simulink library "Navigation_KF_Lib"  (R2016a)
settings: Solver=ode45  StartTime=0.0  StopTime=10.0  RelTol=1e-3
undefined symbols (not defined in the file or in its folder): Accel_Calib_Gain, Accel_Calib_Offset, Mag_Calib_Gain_Vector, Mag_Calib_Offset_Vector
libraries: simulink x5, vrlib x4, aerolibtransform2 x2, aerolibutil x1
(part 1 of 2)
settings Model: Creator=darenlee  LastModifiedBy=sannem
settings DataIOCC: LimitDataPoints=on  SaveFormat=Array
settings DebuggingCC: SolverPrmCheckMsg=warning
settings HardwareCC: ProdBitPerPointer=32  ProdLargestAtomicFloat=None  ProdIntDivRoundTo=Undefined  ProdEndianess=Unspecified  ProdWordSize=32  ProdHWDeviceType=32-bit Generic
settings ModelReferenceCC: PropagateSignalLabelsOutOfModel=off
settings ConfigComp: CovModelRefEnable=Off  CovSFcnEnable=off

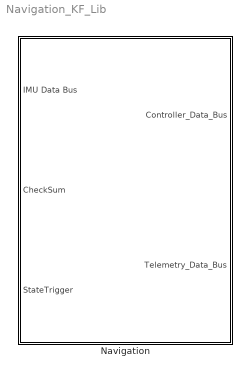
== system Navigation_KF_Lib ==
  Navigation : Subsystem
      mask DialogControl DescTextVar Prompt: Kalman Filter Navigation Implementation

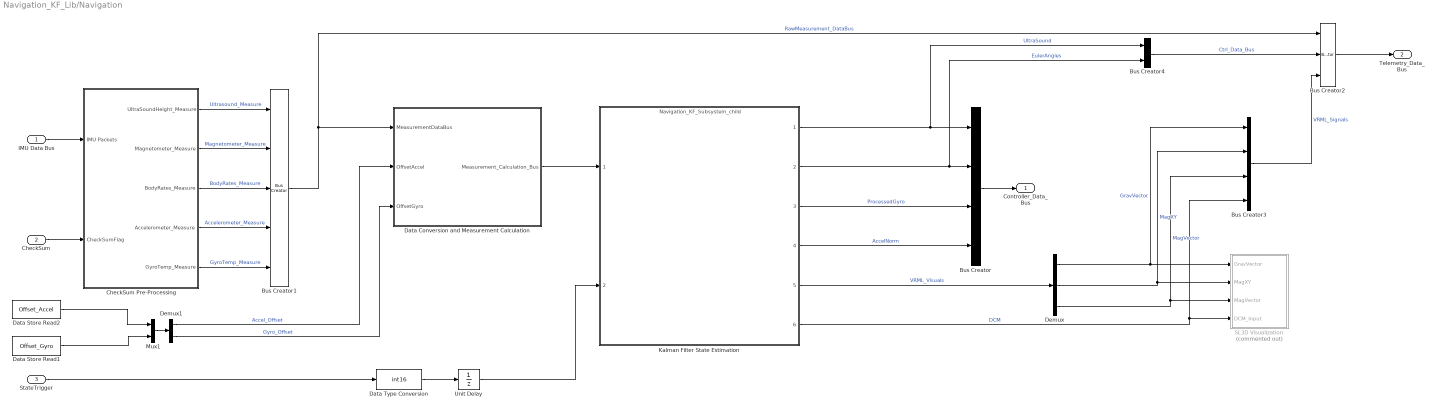
== system Navigation_KF_Lib/Navigation ==
  IMU Data Bus : Inport  OutDataTypeStr=Bus: IMU_Packets
  CheckSum : Inport  Port=2
  StateTrigger : Inport  Port=3  OutDataTypeStr=Enum: Drone_StateModeType
  Bus Creator : BusCreator  Inputs=4
  Bus Creator1 : BusCreator  Inputs=5
  Bus Creator2 : BusCreator  Inputs=3
  Bus Creator3 : BusCreator  Inputs=4
  Bus Creator4 : BusCreator  Inputs=2
  CheckSum Pre-Processing : Subsystem  TreatAsAtomicUnit=on
      settings: RTWSystemCode=Inline
  Data Conversion and Measurement Calculation : Subsystem
  Data Store Read1 : DataStoreRead  DataStoreName=Offset_Gyro
  Data Store Read2 : DataStoreRead  DataStoreName=Offset_Accel
  Data Type Conversion : DataTypeConversion  OutDataTypeStr=int16
  Demux : Demux  Outputs=[3 3 3]
  Demux1 : Demux  Outputs=[2 3]
  Kalman Filter State Estimation : ModelReference  ModelNameDialog=Navigation_KF_Subsystem_child.slx  SimulationMode=Normal  ModelReferenceVersion=1.56
  Mux1 : Mux  Inputs=2
  SL3D Visualization : Subsystem  Commented=on
  Unit Delay : UnitDelay  SampleTime=-1
  Controller_Data_Bus : Outport
  Telemetry_Data_Bus : Outport  Port=2
  wires:
  Bus Creator4/1 -> Bus Creator2/2  "Ctrl_Data_Bus"
  Demux/2 -> SL3D Visualization/2(MagXY), Bus Creator3/2  "MagXY"
  Bus Creator3/1 -> Bus Creator2/3  "VRML_Signals"
  Bus Creator2/1 -> Telemetry_Data_Bus/1
  Data Store Read1/1 -> Mux1/2
  Data Store Read2/1 -> Mux1/1
  Kalman Filter State Estimation/5 -> Demux/1  "VRML_Visuals"
  Kalman Filter State Estimation/2 -> Bus Creator/2, Bus Creator4/2  "EulerAngles"
  Bus Creator/1 -> Controller_Data_Bus/1
  Demux/3 -> SL3D Visualization/3(MagVector), Bus Creator3/3  "MagVector"
  Demux/1 -> SL3D Visualization/1(GravVector), Bus Creator3/1  "GravVector"
  Kalman Filter State Estimation/1 -> Bus Creator/1, Bus Creator4/1  "UltraSound"
  Kalman Filter State Estimation/6 -> SL3D Visualization/4(DCM_Input), Bus Creator3/4  "DCM"
  Data Type Conversion/1 -> Unit Delay/1
  Unit Delay/1 -> Kalman Filter State Estimation/2
  IMU Data Bus/1 -> CheckSum Pre-Processing/1(IMU Packets)
  CheckSum/1 -> CheckSum Pre-Processing/2(CheckSumFlag)
  CheckSum Pre-Processing/1(UltraSoundHeight_Measure) -> Bus Creator1/1  "Ultrasound_Measure"
  CheckSum Pre-Processing/2(Magnetometer_Measure) -> Bus Creator1/2  "Magnetometer_Measure"
  CheckSum Pre-Processing/3(BodyRates_Measure) -> Bus Creator1/3  "BodyRates_Measure"
  CheckSum Pre-Processing/4(Accelerometer_Measure) -> Bus Creator1/4  "Accelerometer_Measure"
  CheckSum Pre-Processing/5(GyroTemp_Measure) -> Bus Creator1/5  "GyroTemp_Measure"
  Bus Creator1/1 -> Data Conversion and Measurement Calculation/1(MeasurementDataBus), Bus Creator2/1  "RawMeasurement_DataBus"
  Mux1/1 -> Demux1/1
  Demux1/1 -> Data Conversion and Measurement Calculation/2(OffsetAccel)  "Accel_Offset"
  Demux1/2 -> Data Conversion and Measurement Calculation/3(OffsetGyro)  "Gyro_Offset"
  StateTrigger/1 -> Data Type Conversion/1
  Data Conversion and Measurement Calculation/1(Measurement_Calculation_Bus) -> Kalman Filter State Estimation/1
  Kalman Filter State Estimation/3 -> Bus Creator/3  "ProcessedGyro"
  Kalman Filter State Estimation/4 -> Bus Creator/4  "AccelNorm"

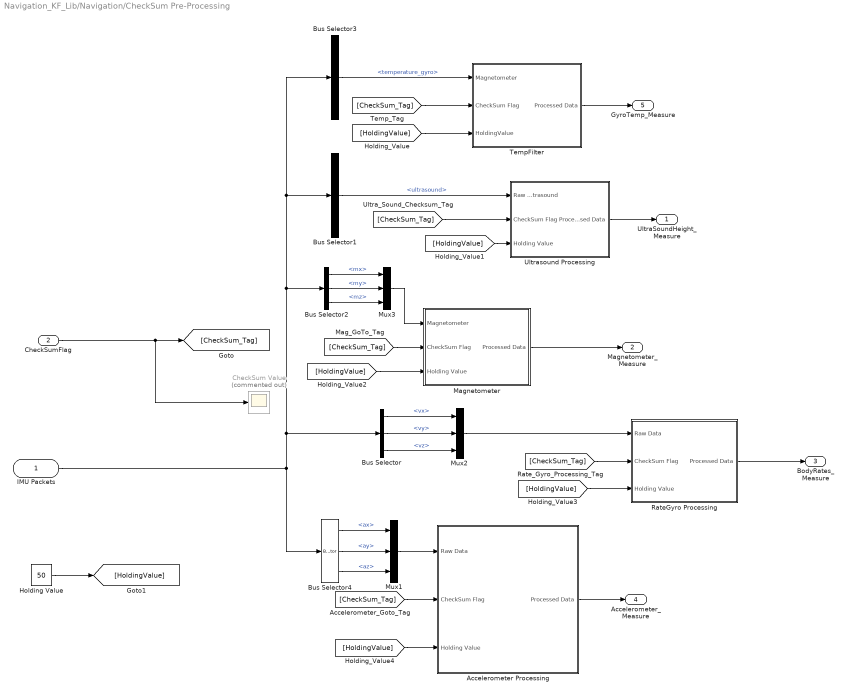
== system Navigation_KF_Lib/Navigation/CheckSum Pre-Processing ==
  IMU Packets : Inport
  CheckSumFlag : Inport  Port=2
  Accelerometer Processing : Subsystem
  Bus Selector : BusSelector  OutputSignals=vx,vy,vz
  Bus Selector1 : BusSelector  OutputSignals=ultrasound
  Bus Selector2 : BusSelector  OutputSignals=mx,my,mz
  Bus Selector3 : BusSelector  OutputSignals=temperature_gyro
  Bus Selector4 : BusSelector  OutputSignals=ax,ay,az
  CheckSum Value : Scope  Commented=on
  Holding Value : Constant  Value=50
  Magnetometer : Subsystem
  Mux1 : Mux  Inputs=3
  Mux2 : Mux  Inputs=3
  Mux3 : Mux  Inputs=3
  RateGyro Processing : Subsystem
  TempFilter : Subsystem
  Ultrasound Processing : Subsystem
  UltraSoundHeight_Measure : Outport
  Magnetometer_Measure : Outport  Port=2
  BodyRates_Measure : Outport  Port=3
  Accelerometer_Measure : Outport  Port=4
  GyroTemp_Measure : Outport  Port=5
  wires:
  Bus Selector1/1 -> Ultrasound Processing/1(Raw Ultrasound)  "<ultrasound>"
  CheckSumFlag/1 -> [CheckSum_Tag], CheckSum Value/1
  IMU Packets/1 -> Bus Selector/1, Bus Selector3/1, Bus Selector1/1, Bus Selector2/1, Bus Selector4/1
  Bus Selector4/1 -> Mux1/1  "<ax>"
  Bus Selector4/2 -> Mux1/2  "<ay>"
  Bus Selector4/3 -> Mux1/3  "<az>"
  Mux1/1 -> Accelerometer Processing/1(Raw Data)
  [CheckSum_Tag] -> Ultrasound Processing/2(CheckSum Flag)
  Accelerometer Processing/1(Processed Data) -> Accelerometer_Measure/1
  Mux2/1 -> RateGyro Processing/1(Raw Data)
  [CheckSum_Tag] -> RateGyro Processing/2(CheckSum Flag)
  RateGyro Processing/1(Processed Data) -> BodyRates_Measure/1
  Bus Selector2/1 -> Mux3/1  "<mx>"
  Bus Selector2/2 -> Mux3/2  "<my>"
  Bus Selector2/3 -> Mux3/3  "<mz>"
  [CheckSum_Tag] -> Magnetometer/2(CheckSum Flag)
  Magnetometer/1(Processed Data) -> Magnetometer_Measure/1
  [CheckSum_Tag] -> Accelerometer Processing/2(CheckSum Flag)
  Ultrasound Processing/1(Processed Data) -> UltraSoundHeight_Measure/1
  Bus Selector/1 -> Mux2/1  "<vx>"
  Bus Selector/2 -> Mux2/2  "<vy>"
  Bus Selector/3 -> Mux2/3  "<vz>"
  Bus Selector3/1 -> TempFilter/1(Magnetometer)  "<temperature_gyro>"
  TempFilter/1(Processed Data) -> GyroTemp_Measure/1
  [CheckSum_Tag] -> TempFilter/2(CheckSum Flag)
  [HoldingValue] -> TempFilter/3(HoldingValue)
  [HoldingValue] -> Ultrasound Processing/3(Holding Value)
  [HoldingValue] -> Magnetometer/3(Holding Value)
  [HoldingValue] -> RateGyro Processing/3(Holding Value)
  [HoldingValue] -> Accelerometer Processing/3(Holding Value)
  Holding Value/1 -> [HoldingValue]
  Mux3/1 -> Magnetometer/1(Magnetometer)

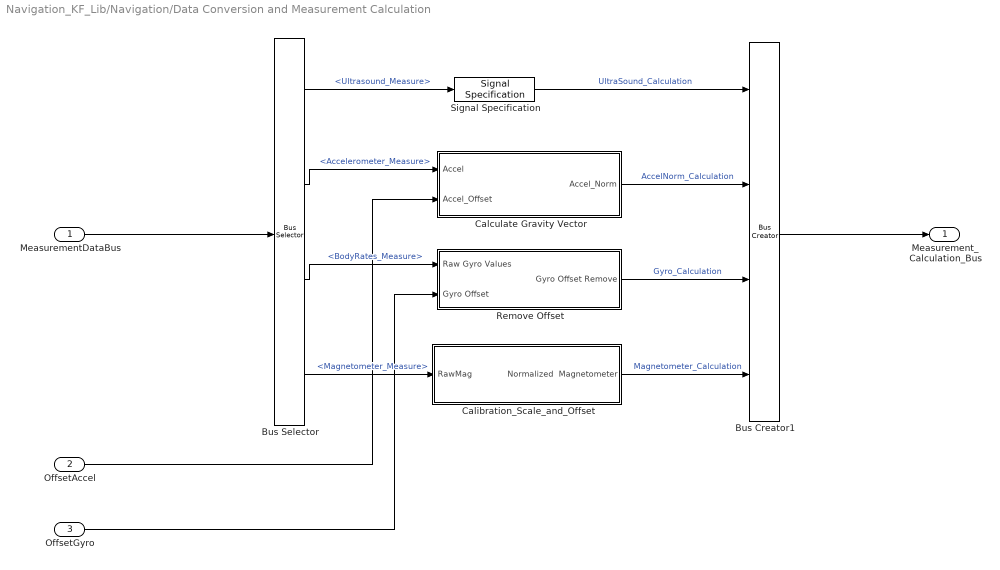
== system Navigation_KF_Lib/Navigation/Data Conversion and Measurement Calculation ==
  MeasurementDataBus : Inport
  OffsetAccel : Inport  Port=2
  OffsetGyro : Inport  Port=3
  Bus Creator1 : BusCreator  Inputs=4
  Bus Selector : BusSelector  OutputSignals=Ultrasound_Measure,Accelerometer_Measure,BodyRates_Measure,Magnetometer_Measure
  Calculate Gravity Vector : Subsystem
  Calibration_Scale_and_Offset : Subsystem
  Remove Offset : Subsystem
  Signal Specification : SignalSpecification
  Measurement_Calculation_Bus : Outport
  wires:
  Bus Selector/2 -> Calculate Gravity Vector/1(Accel)  "<Accelerometer_Measure>"
  Bus Creator1/1 -> Measurement_Calculation_Bus/1
  Calculate Gravity Vector/1(Accel_Norm) -> Bus Creator1/2  "AccelNorm_Calculation"
  Signal Specification/1 -> Bus Creator1/1  "UltraSound_Calculation"
  Remove Offset/1(Gyro Offset Remove) -> Bus Creator1/3  "Gyro_Calculation"
  Calibration_Scale_and_Offset/1(Normalized  Magnetometer) -> Bus Creator1/4  "Magnetometer_Calculation"
  Bus Selector/1 -> Signal Specification/1  "<Ultrasound_Measure>"
  Bus Selector/3 -> Remove Offset/1(Raw Gyro Values)  "<BodyRates_Measure>"
  OffsetGyro/1 -> Remove Offset/2(Gyro Offset)
  OffsetAccel/1 -> Calculate Gravity Vector/2(Accel_Offset)
  Bus Selector/4 -> Calibration_Scale_and_Offset/1(RawMag)  "<Magnetometer_Measure>"
  MeasurementDataBus/1 -> Bus Selector/1

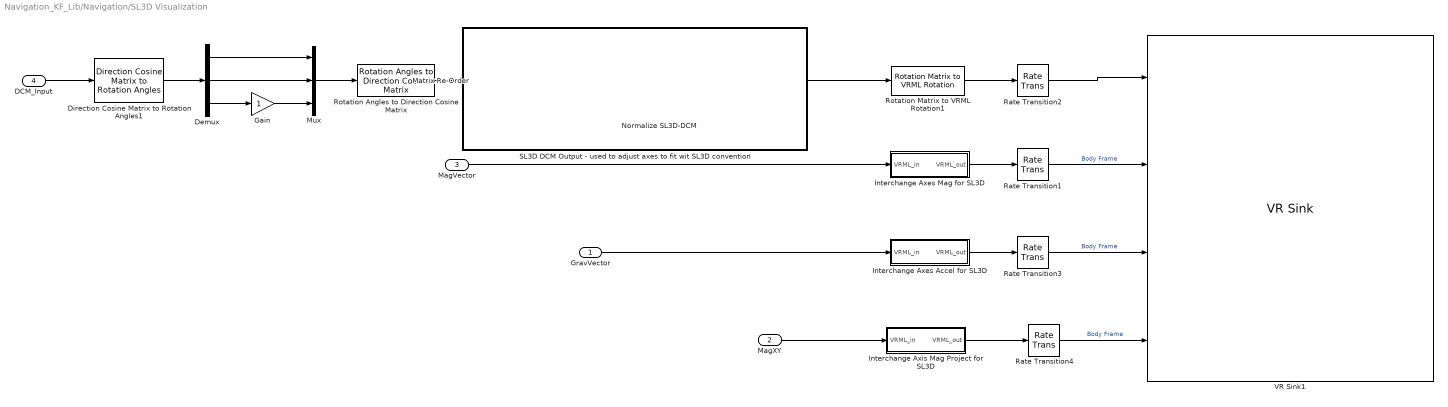
== system Navigation_KF_Lib/Navigation/SL3D Visualization ==
  GravVector : Inport
  MagXY : Inport  Port=2
  MagVector : Inport  Port=3
  DCM_Input : Inport  Port=4
  Demux : Demux  Outputs=3
  Direction Cosine Matrix to Rotation Angles1 : aerolibtransform2/Direction Cosine Matrix to Rotation Angles  rotationOrder=XYZ  lim=ZeroR3
      settings: AttributesFormatString=Rotation Order: %<rotationOrder>
  Gain : Gain  OutDataTypeStr=Inherit: Same as input
  "Interchange Axes Accel for SL3D " : Subsystem
  "Interchange Axes Mag for SL3D " : Subsystem
  Interchange Axis Mag Project for SL3D : Subsystem
  Matrix Re-Order : MATLAB Function  TreatAsAtomicUnit=on
  Mux : Mux  Inputs=3
  Normalize SL3D-DCM : Subsystem  TreatAsAtomicUnit=on
  Rate Transition{1..4} (4 alike) : RateTransition
  Rotation Angles to Direction Cosine Matrix : aerolibtransform2/Rotation Angles to Direction Cosine Matrix  rotationOrder=XYZ
  Rotation Matrix to VRML Rotation1 : vrlib/Utilities/Rotation Matrix to VRML Rotation  maxzero=1e-12
  SL3D DCM Output - used to adjust axes to fit wit SL3D convention : Subsystem
  VR Sink1 : vrlib/VR Sink  InstantiateOnLoad=on  SampleTime=0.02  ViewEnable=on  RemoteChange=off  RemoteView=off  FieldsWritten=Plane.rotation.4.1.1.double#mag_point.translation.3.1.1.double#grav_point.translation.3.1.1.double#mag_projection_point.translation.3.1.1.double  WorldFileName=vrml8_grav_2.WRL  AutoView=off  VideoDimensions=[]  AllowVariableSize=off
  wires:
  Rotation Matrix to VRML Rotation1/1 -> Rate Transition2/1
  "Interchange Axes Accel for SL3D "/1(VRML_out) -> Rate Transition3/1
  DCM_Input/1 -> Direction Cosine Matrix to Rotation Angles1/1
  GravVector/1 -> "Interchange Axes Accel for SL3D "/1(VRML_in)
  Matrix Re-Order/1(M_out) -> Normalize SL3D-DCM/1(DCM)
  Normalize SL3D-DCM/1(DCM_normalized) -> Rotation Matrix to VRML Rotation1/1
  Direction Cosine Matrix to Rotation Angles1/1 -> Demux/1
  Demux/1 -> Mux/1
  Demux/2 -> Mux/2
  Demux/3 -> Gain/1
  Gain/1 -> Mux/3
  Mux/1 -> Rotation Angles to Direction Cosine Matrix/1
  "Interchange Axes Mag for SL3D "/1(VRML_out) -> Rate Transition1/1
  MagVector/1 -> "Interchange Axes Mag for SL3D "/1(VRML_in)
  Rotation Angles to Direction Cosine Matrix/1 -> Matrix Re-Order/1(M_in)
  Interchange Axis Mag Project for SL3D/1(VRML_out) -> Rate Transition4/1
  Rate Transition4/1 -> VR Sink1/4  "Body Frame"
  Rate Transition3/1 -> VR Sink1/3  "Body Frame"
  Rate Transition1/1 -> VR Sink1/2  "Body Frame"
  Rate Transition2/1 -> VR Sink1/1
  MagXY/1 -> Interchange Axis Mag Project for SL3D/1(VRML_in)

== system Navigation_KF_Lib/Navigation/CheckSum Pre-Processing/Accelerometer Processing ==
  Raw Data : Inport
  CheckSum Flag : Inport  Port=2
  Holding Value : Inport  Port=3
  Calculate Accel Data : Subsystem  Commented=through
  CheckSum Correction : Subsystem
  Processed Data : Outport
  wires:
  CheckSum Flag/1 -> CheckSum Correction/2(CheckSumFlag)
  Raw Data/1 -> Calculate Accel Data/1(Raw Accel Data)
  CheckSum Correction/1(Pre-Processed Height) -> Processed Data/1
  Calculate Accel Data/1(Processed Accel Data) -> CheckSum Correction/1(CalculatedData)
  Holding Value/1 -> CheckSum Correction/3(Holding Value)

== system Navigation_KF_Lib/Navigation/CheckSum Pre-Processing/Magnetometer ==
  Magnetometer : Inport
  CheckSum Flag : Inport  Port=2
  Holding Value : Inport  Port=3
  CheckSum Correction : Subsystem
  Process Raw Mag Data : Subsystem  Commented=through
  Processed Data : Outport
  wires:
  CheckSum Flag/1 -> CheckSum Correction/2(CheckSumFlag)
  CheckSum Correction/1(Pre-Processed Data) -> Processed Data/1
  Magnetometer/1 -> Process Raw Mag Data/1(Magnetometer)
  Process Raw Mag Data/1(ProcessedData) -> CheckSum Correction/1(CalculatedData)
  Holding Value/1 -> CheckSum Correction/3(Holding Value)

== system Navigation_KF_Lib/Navigation/CheckSum Pre-Processing/RateGyro Processing ==
  Raw Data : Inport
  CheckSum Flag : Inport  Port=2
  Holding Value : Inport  Port=3
  CheckSum Correction : Subsystem
  Process Data : Subsystem  Commented=through
  Processed Data : Outport
  wires:
  CheckSum Flag/1 -> CheckSum Correction/2(CheckSumFlag)
  CheckSum Correction/1(Pre-Processed Height) -> Processed Data/1
  Raw Data/1 -> Process Data/1(Raw Data)
  Process Data/1(Processed Data) -> CheckSum Correction/1(CalculatedData)
  Holding Value/1 -> CheckSum Correction/3(Holding Value)

== system Navigation_KF_Lib/Navigation/CheckSum Pre-Processing/TempFilter ==
  Magnetometer : Inport
  CheckSum Flag : Inport  Port=2
  HoldingValue : Inport  Port=3
  CheckSum Correction : Subsystem
  Process Raw Mag Data : Subsystem  Commented=through
  Processed Data : Outport
  wires:
  CheckSum Flag/1 -> CheckSum Correction/2(CheckSumFlag)
  CheckSum Correction/1(Pre-Processed Data) -> Processed Data/1
  Magnetometer/1 -> Process Raw Mag Data/1(Magnetometer)
  Process Raw Mag Data/1(ProcessedData) -> CheckSum Correction/1(CalculatedData)
  HoldingValue/1 -> CheckSum Correction/3(Holding Value)

== system Navigation_KF_Lib/Navigation/CheckSum Pre-Processing/Ultrasound Processing ==
  note: '192.168.1.1' 1 17725
  Raw Ultrasound : Inport
  CheckSum Flag : Inport  Port=2
  Holding Value : Inport  Port=3
  CheckSum Correction : Subsystem
  Data Type Conversion1 : DataTypeConversion
  Delay1 : Delay  DelayLength=1  InitialCondition=0
  Height Calculation : MATLAB Function  TreatAsAtomicUnit=on
  Saturation1 : Saturate  UpperLimit=100e3  LowerLimit=0
  Processed Data : Outport
  wires:
  Delay1/1 -> Height Calculation/2(z_1)
  Data Type Conversion1/1 -> Height Calculation/1(u)
  Height Calculation/2(prev_good_height) -> Delay1/1
  Raw Ultrasound/1 -> Data Type Conversion1/1
  Height Calculation/1(y) -> CheckSum Correction/1(CalculatedData)
  CheckSum Flag/1 -> CheckSum Correction/2(CheckSumFlag)
  CheckSum Correction/1(Pre-Processed Height) -> Saturation1/1
  Saturation1/1 -> Processed Data/1
  Holding Value/1 -> CheckSum Correction/3(Holding Value)

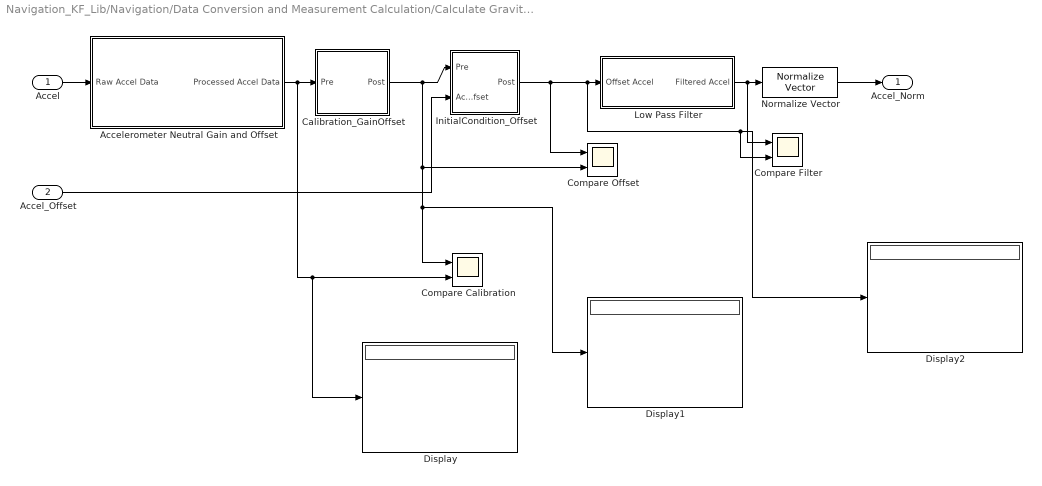
== system Navigation_KF_Lib/Navigation/Data Conversion and Measurement Calculation/Calculate Gravity Vector ==
  Accel : Inport
  Accel_Offset : Inport  Port=2
  Accelerometer Neutral Gain and Offset : Subsystem
  Calibration_GainOffset : Subsystem
  Compare Calibration : Scope  NumInputPorts=2
  Compare Filter : Scope  NumInputPorts=2
  Compare Offset : Scope  NumInputPorts=2
  Display : Display
  Display1 : Display
  Display2 : Display
  InitialCondition_Offset : Subsystem
  Low Pass Filter : Subsystem
  Normalize Vector : vrlib/Utilities/Normalize Vector  maxzero=0
  Accel_Norm : Outport
  wires:
  Normalize Vector/1 -> Accel_Norm/1
  Accel/1 -> Accelerometer Neutral Gain and Offset/1(Raw Accel Data)
  InitialCondition_Offset/1(Post) -> Compare Offset/1, Compare Filter/2, Display2/1, Low Pass Filter/1(Offset Accel)
  Low Pass Filter/1(Filtered Accel) -> Compare Filter/1, Normalize Vector/1
  Calibration_GainOffset/1(Post) -> InitialCondition_Offset/1(Pre), Compare Calibration/1, Display1/1, Compare Offset/2
  Accelerometer Neutral Gain and Offset/1(Processed Accel Data) -> Calibration_GainOffset/1(Pre), Compare Calibration/2, Display/1
  Accel_Offset/1 -> InitialCondition_Offset/2(Accel_Offset)

== system Navigation_KF_Lib/Navigation/Data Conversion and Measurement Calculation/Calibration_Scale_and_Offset ==
  RawMag : Inport
  Normalize Vector : vrlib/Utilities/Normalize Vector  maxzero=0
  Process Raw Mag Data : Subsystem  Variant=on  OverrideUsingVariant=TempVariantA
  Normalized  Magnetometer : Outport
  wires:
  Normalize Vector/1 -> Normalized  Magnetometer/1
  RawMag/1 -> Process Raw Mag Data/1(Magnetometer)
  Process Raw Mag Data/1(MagVector) -> Normalize Vector/1

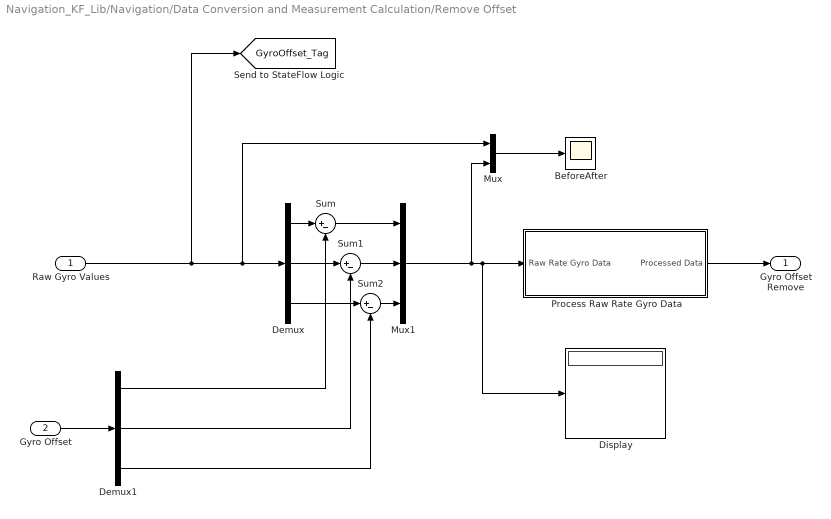
== system Navigation_KF_Lib/Navigation/Data Conversion and Measurement Calculation/Remove Offset ==
  Raw Gyro Values : Inport
  Gyro Offset : Inport  Port=2
  BeforeAfter : Scope
  Demux : Demux  Outputs=3
  Demux1 : Demux  Outputs=3
  Display : Display
  Mux : Mux  Inputs=2
  Mux1 : Mux  Inputs=3
  Process Raw Rate Gyro Data : Subsystem
  Sum : Sum  Inputs=|+-
  Sum1 : Sum  Inputs=|+-
  Sum2 : Sum  Inputs=|+-
  Gyro Offset Remove : Outport
  tag scope: GyroOffset_Tag=global
  wires:
  Sum/1 -> Mux1/1
  Sum2/1 -> Mux1/3
  Demux/3 -> Sum2/1
  Sum1/1 -> Mux1/2
  Demux/1 -> Sum/1
  Demux/2 -> Sum1/1
  Demux1/1 -> Sum/2
  Demux1/2 -> Sum1/2
  Demux1/3 -> Sum2/2
  Mux1/1 -> Mux/2, Display/1, Process Raw Rate Gyro Data/1(Raw Rate Gyro Data)
  Gyro Offset/1 -> Demux1/1
  Raw Gyro Values/1 -> [GyroOffset_Tag], Mux/1, Demux/1
  Mux/1 -> BeforeAfter/1
  Process Raw Rate Gyro Data/1(Processed Data) -> Gyro Offset Remove/1

== system Navigation_KF_Lib/Navigation/SL3D Visualization/Interchange Axes Accel for SL3D  ==
  VRML_in : Inport
  Demux1 : Demux  Outputs=3
  Gain1 : Gain  Gain=3
  Gain2 : Gain
  Gain3 : Gain
  Mux2 : Mux  Inputs=3
  VRML_out : Outport
  wires:
  Gain1/1 -> Demux1/1
  Demux1/1 -> Gain3/1
  Demux1/3 -> Mux2/2
  Gain2/1 -> Mux2/1
  Gain3/1 -> Mux2/3
  Mux2/1 -> VRML_out/1
  Demux1/2 -> Gain2/1
  VRML_in/1 -> Gain1/1

== system Navigation_KF_Lib/Navigation/SL3D Visualization/Interchange Axes Mag for SL3D  ==
  VRML_in : Inport
  Home Drone : Subsystem
  Subsystem : Subsystem  Commented=on
  Work Drone : Subsystem
  Work Drone - supposed work drone .. not really : Subsystem
  VRML_out : Outport
  wires:
  VRML_in/1 -> Work Drone/1(In1), Home Drone/1(In1)
  Work Drone/1(Out1) -> VRML_out/1

== system Navigation_KF_Lib/Navigation/SL3D Visualization/Interchange Axis Mag Project for SL3D ==
  VRML_in : Inport
  Demux1 : Demux  Outputs=3
  Gain2 : Gain
  Gain3 : Gain
  Mux2 : Mux  Inputs=3
  VRML_out : Outport
  wires:
  VRML_in/1 -> Demux1/1
  Demux1/1 -> Gain3/1
  Demux1/3 -> Mux2/2
  Gain2/1 -> Mux2/1
  Gain3/1 -> Mux2/3
  Mux2/1 -> VRML_out/1
  Demux1/2 -> Gain2/1

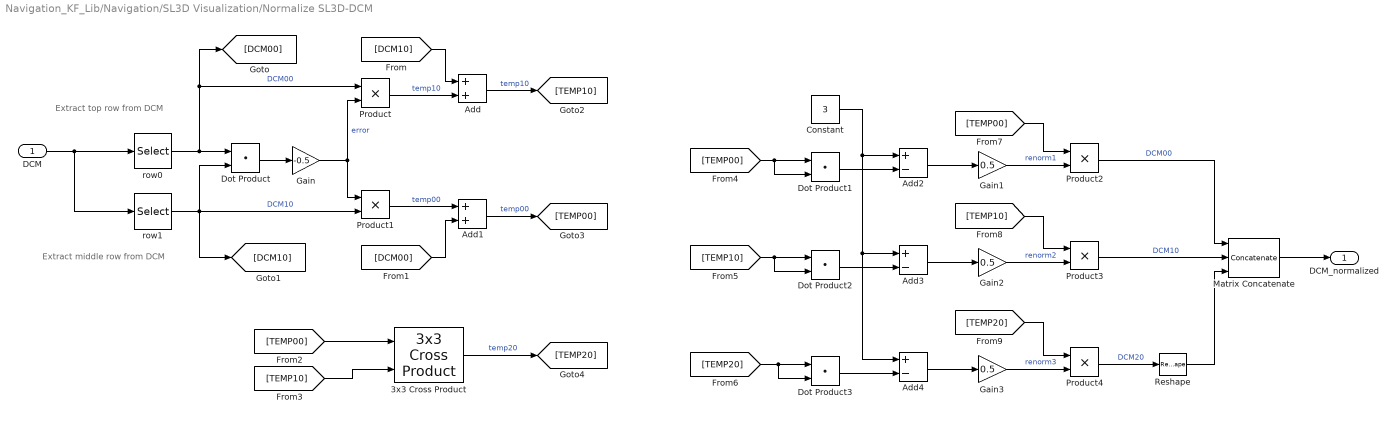
== system Navigation_KF_Lib/Navigation/SL3D Visualization/Normalize SL3D-DCM ==
  note: Extract middle row from DCM
  note: Extract top row from DCM
  DCM : Inport  OutDataTypeStr=double  PortDimensions=[3,3]
  3x3 Cross Product : aerolibutil/3x3 Cross Product
  Add : Sum
  Add1 : Sum
  Add2 : Sum  Inputs=+-
  Add3 : Sum  Inputs=+-
  Add4 : Sum  Inputs=+-
  Constant : Constant  Value=3  OutDataTypeStr=double  SampleTime=-1
  Dot Product{,1..3} (4 alike) : DotProduct  InputSameDT=on  OutDataTypeStr=Inherit: Inherit via internal rule
  Gain : Gain  Gain=-0.5
  Gain1 : Gain  Gain=0.5  OutDataTypeStr=single
  Gain2 : Gain  Gain=0.5  OutDataTypeStr=single
  Gain3 : Gain  Gain=0.5  OutDataTypeStr=single
  Matrix Concatenate : Concatenate  NumInputs=3  Mode=Multidimensional array
  Product{,1..4} (5 alike) : Product  RndMeth=Zero
  Reshape : Reshape  OutputDimensionality=Row vector (2-D)
  row0 : Selector  NumberOfDimensions=2  IndexMode=Zero-based  InputPortWidth=3  IndexOptions=Index vector (dialog),Index vector (dialog)  Indices=0,[0:2]  OutputSizes=1,1
  row1 : Selector  NumberOfDimensions=2  IndexMode=Zero-based  InputPortWidth=3  IndexOptions=Index vector (dialog),Index vector (dialog)  Indices=1,[0:2]  OutputSizes=1,1
  DCM_normalized : Outport  OutDataTypeStr=double
  wires:
  Reshape/1 -> Matrix Concatenate/3
  Matrix Concatenate/1 -> DCM_normalized/1
  Product4/1 -> Reshape/1  "DCM20"
  Product3/1 -> Matrix Concatenate/2  "DCM10"
  Product2/1 -> Matrix Concatenate/1  "DCM00"
  [TEMP20] -> Product4/1
  [TEMP10] -> Product3/1
  [TEMP00] -> Product2/1
  Dot Product3/1 -> Add4/2
  Gain3/1 -> Product4/2  "renorm3"
  Add4/1 -> Gain3/1
  Dot Product2/1 -> Add3/2
  Gain2/1 -> Product3/2  "renorm2"
  Add3/1 -> Gain2/1
  Gain1/1 -> Product2/2  "renorm1"
  Add2/1 -> Gain1/1
  Constant/1 -> Add3/1, Add4/1, Add2/1
  Dot Product1/1 -> Add2/2
  [TEMP20] -> Dot Product3/2, Dot Product3/1
  [TEMP10] -> Dot Product2/2, Dot Product2/1
  [TEMP00] -> Dot Product1/2, Dot Product1/1
  [TEMP10] -> 3x3 Cross Product/2
  [TEMP00] -> 3x3 Cross Product/1
  3x3 Cross Product/1 -> [TEMP20]  "temp20"
  Add1/1 -> [TEMP00]  "temp00"
  Add/1 -> [TEMP10]  "temp10"
  [DCM00] -> Add1/2
  [DCM10] -> Add/1
  Product1/1 -> Add1/1  "temp00"
  Product/1 -> Add/2  "temp10"
  Gain/1 -> Product1/1, Product/2  "error"
  Dot Product/1 -> Gain/1
  row1/1 -> [DCM10], Product1/2, Dot Product/2  "DCM10"
  row0/1 -> [DCM00], Product/1, Dot Product/1  "DCM00"
  DCM/1 -> row1/1, row0/1

== system Navigation_KF_Lib/Navigation/SL3D Visualization/SL3D DCM Output - used to adjust axes to fit wit SL3D convention ==

== system Navigation_KF_Lib/Navigation/CheckSum Pre-Processing/Accelerometer Processing/Calculate Accel Data ==
  Raw Accel Data : Inport
  Bias : Constant  Value=[0 4096 4096]
  Gain : Gain  Gain=[0.001953125, 0.001953125, 0.001953125]
  Neutral Bias : Constant  Value=[2048 2048 2048]
  Sum : Sum  Inputs=|-+
  Sum1 : Sum  Inputs=|+-
  Processed Accel Data : Outport
  wires:
  Raw Accel Data/1 -> Sum/1
  Sum1/1 -> Gain/1
  Gain/1 -> Processed Accel Data/1
  Sum/1 -> Sum1/1
  Neutral Bias/1 -> Sum1/2
  Bias/1 -> Sum/2

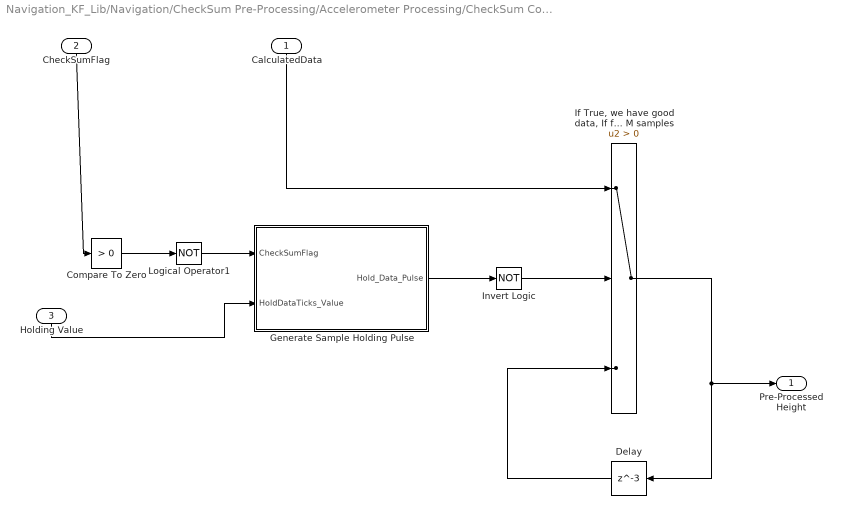
== system Navigation_KF_Lib/Navigation/CheckSum Pre-Processing/Accelerometer Processing/CheckSum Correction ==
  CalculatedData : Inport
  CheckSumFlag : Inport  Port=2
  Holding Value : Inport  Port=3
  Compare To Zero : simulink/Logic and Bit Operations/Compare To Zero  relop=>  OutDataTypeStr=boolean
  Delay : Delay  DelayLength=3  InitialCondition=0
  Generate Sample Holding Pulse : Subsystem
  "If True, we have good data, If false, we have bad data, With bad data, use previous good data from N samples ago and hold it on that value for M samples" : Switch  Criteria=u2 > Threshold
  Invert Logic : Logic  Operator=NOT  AllPortsSameDT=off  OutDataTypeStr=boolean
  Logical Operator1 : Logic  Operator=NOT  AllPortsSameDT=off  OutDataTypeStr=boolean
  Pre-Processed Height : Outport
  wires:
  CheckSumFlag/1 -> Compare To Zero/1
  CalculatedData/1 -> "If True, we have good data, If false, we have bad data, With bad data, use previous good data from N samples ago and hold it on that value for M samples"/1
  "If True, we have good data, If false, we have bad data, With bad data, use previous good data from N samples ago and hold it on that value for M samples"/1 -> Pre-Processed Height/1, Delay/1
  Delay/1 -> "If True, we have good data, If false, we have bad data, With bad data, use previous good data from N samples ago and hold it on that value for M samples"/3
  Compare To Zero/1 -> Logical Operator1/1
  Generate Sample Holding Pulse/1(Hold_Data_Pulse) -> Invert Logic/1
  Logical Operator1/1 -> Generate Sample Holding Pulse/1(CheckSumFlag)
  Invert Logic/1 -> "If True, we have good data, If false, we have bad data, With bad data, use previous good data from N samples ago and hold it on that value for M samples"/2
  Holding Value/1 -> Generate Sample Holding Pulse/2(HoldDataTicks_Value)

== system Navigation_KF_Lib/Navigation/CheckSum Pre-Processing/Magnetometer/CheckSum Correction ==
  CalculatedData : Inport
  CheckSumFlag : Inport  Port=2
  Holding Value : Inport  Port=3
  Compare To Zero : simulink/Logic and Bit Operations/Compare To Zero  relop=>  OutDataTypeStr=boolean
  Delay : Delay  DelayLength=3  InitialCondition=0
  Generate Sample Holding Pulse : Subsystem
  "If True, we have good data, If false, we have bad data, With bad data, use previous good data from N samples ago and hold it on that value for M samples" : Switch  Criteria=u2 > Threshold
  Invert Logic : Logic  Operator=NOT  AllPortsSameDT=off  OutDataTypeStr=boolean
  Logical Operator1 : Logic  Operator=NOT  AllPortsSameDT=off  OutDataTypeStr=boolean
  Pre-Processed Data : Outport
  wires:
  CheckSumFlag/1 -> Compare To Zero/1
  CalculatedData/1 -> "If True, we have good data, If false, we have bad data, With bad data, use previous good data from N samples ago and hold it on that value for M samples"/1
  "If True, we have good data, If false, we have bad data, With bad data, use previous good data from N samples ago and hold it on that value for M samples"/1 -> Pre-Processed Data/1, Delay/1
  Delay/1 -> "If True, we have good data, If false, we have bad data, With bad data, use previous good data from N samples ago and hold it on that value for M samples"/3
  Compare To Zero/1 -> Logical Operator1/1
  Generate Sample Holding Pulse/1(Hold_Data_Pulse) -> Invert Logic/1
  Logical Operator1/1 -> Generate Sample Holding Pulse/1(CheckSumFlag)
  Invert Logic/1 -> "If True, we have good data, If false, we have bad data, With bad data, use previous good data from N samples ago and hold it on that value for M samples"/2
  Holding Value/1 -> Generate Sample Holding Pulse/2(HoldDataTicks_Value)

== system Navigation_KF_Lib/Navigation/CheckSum Pre-Processing/Magnetometer/Process Raw Mag Data ==
  note: magnetometer[ 0 ] = - ( float ) navdata.mx ;
      | magnetometer[ 1 ] = ( float ) navdata.my ;
      | magnetometer[ 2 ] = - ( float ) navdata.mz ;
      | const float Sensitivity[ 3 ] = { 0.0071492608 , 0.0070882491 , 0.0074057781 } ;
      | const float Neutral[ 3 ] = { 118.0 , - 65.0 , 110.0 } ;
  Magnetometer : Inport
  Bias : Constant  Value=[ 118.0, -65.0, 110.0 ]
  Sum : Sum  Inputs=|+-
  postGain : Gain  Gain=[0.0071492608, 0.0070882491, 0.0074057781]
  preGain : Gain  Gain=[-1 1 -1]
  ProcessedData : Outport
  wires:
  postGain/1 -> ProcessedData/1
  Magnetometer/1 -> preGain/1
  Sum/1 -> postGain/1
  preGain/1 -> Sum/1
  Bias/1 -> Sum/2

== system Navigation_KF_Lib/Navigation/CheckSum Pre-Processing/RateGyro Processing/CheckSum Correction ==
  CalculatedData : Inport
  CheckSumFlag : Inport  Port=2
  Holding Value : Inport  Port=3
  Compare To Zero : simulink/Logic and Bit Operations/Compare To Zero  relop=>  OutDataTypeStr=boolean
  Delay : Delay  DelayLength=3  InitialCondition=0
  Generate Sample Holding Pulse : Subsystem
  "If True, we have good data, If false, we have bad data, With bad data, use previous good data from N samples ago and hold it on that value for M samples" : Switch  Criteria=u2 > Threshold
  Invert Logic : Logic  Operator=NOT  AllPortsSameDT=off  OutDataTypeStr=boolean
  Logical Operator1 : Logic  Operator=NOT  AllPortsSameDT=off  OutDataTypeStr=boolean
  Pre-Processed Height : Outport
  wires:
  CheckSumFlag/1 -> Compare To Zero/1
  CalculatedData/1 -> "If True, we have good data, If false, we have bad data, With bad data, use previous good data from N samples ago and hold it on that value for M samples"/1
  "If True, we have good data, If false, we have bad data, With bad data, use previous good data from N samples ago and hold it on that value for M samples"/1 -> Pre-Processed Height/1, Delay/1
  Delay/1 -> "If True, we have good data, If false, we have bad data, With bad data, use previous good data from N samples ago and hold it on that value for M samples"/3
  Compare To Zero/1 -> Logical Operator1/1
  Generate Sample Holding Pulse/1(Hold_Data_Pulse) -> Invert Logic/1
  Logical Operator1/1 -> Generate Sample Holding Pulse/1(CheckSumFlag)
  Invert Logic/1 -> "If True, we have good data, If false, we have bad data, With bad data, use previous good data from N samples ago and hold it on that value for M samples"/2
  Holding Value/1 -> Generate Sample Holding Pulse/2(HoldDataTicks_Value)

== system Navigation_KF_Lib/Navigation/CheckSum Pre-Processing/RateGyro Processing/Process Data ==
  note: const float Sensitivity[ 3 ] = { 0.0609 , 0.0609 , 0.0609 } ;
      | const float Neutral[ 3 ] = { 0.0 , 0.0 , 0.0 } ;
      | const int16_t Offset[ 3 ] = { - 73 , 14 , - 13 } ;
      | const int16_t Noises[ 3 ] = { 35 , 35 , 15 } ;
      |
      | int16_t vRaws[ 3 ] = {
      | Navdata :: IMU :: Gyroscope :: getRawX (),
      | Navdata :: IMU :: Gyroscope :: getRawY (),
      | Navdata :: IMU :: Gyroscope :: getRawZ ()
      | } ;
      |
      | gyroscope[i] = vRaws[i] * Gyroscope :: Sensitivity[i] * M_PI / 180.0 ;
  Raw Data : Inport
  Constant : Constant  Value=[0.0, 0.0, 0.0]
  Gain : Gain  Gain=[0.0609, 0.0609, 0.0609]
  Sum : Sum  Inputs=|++
  Processed Data : Outport
  wires:
  Sum/1 -> Gain/1
  Gain/1 -> Processed Data/1
  Constant/1 -> Sum/2
  Raw Data/1 -> Sum/1

== system Navigation_KF_Lib/Navigation/CheckSum Pre-Processing/TempFilter/CheckSum Correction ==
  CalculatedData : Inport
  CheckSumFlag : Inport  Port=2
  Holding Value : Inport  Port=3
  Compare To Zero : simulink/Logic and Bit Operations/Compare To Zero  relop=>  OutDataTypeStr=boolean
  Delay : Delay  DelayLength=3  InitialCondition=0
  Generate Sample Holding Pulse : Subsystem
  "If True, we have good data, If false, we have bad data, With bad data, use previous good data from N samples ago and hold it on that value for M samples" : Switch  Criteria=u2 > Threshold
  Invert Logic : Logic  Operator=NOT  AllPortsSameDT=off  OutDataTypeStr=boolean
  Logical Operator1 : Logic  Operator=NOT  AllPortsSameDT=off  OutDataTypeStr=boolean
  Pre-Processed Data : Outport
  wires:
  CheckSumFlag/1 -> Compare To Zero/1
  CalculatedData/1 -> "If True, we have good data, If false, we have bad data, With bad data, use previous good data from N samples ago and hold it on that value for M samples"/1
  "If True, we have good data, If false, we have bad data, With bad data, use previous good data from N samples ago and hold it on that value for M samples"/1 -> Pre-Processed Data/1, Delay/1
  Delay/1 -> "If True, we have good data, If false, we have bad data, With bad data, use previous good data from N samples ago and hold it on that value for M samples"/3
  Compare To Zero/1 -> Logical Operator1/1
  Generate Sample Holding Pulse/1(Hold_Data_Pulse) -> Invert Logic/1
  Logical Operator1/1 -> Generate Sample Holding Pulse/1(CheckSumFlag)
  Invert Logic/1 -> "If True, we have good data, If false, we have bad data, With bad data, use previous good data from N samples ago and hold it on that value for M samples"/2
  Holding Value/1 -> Generate Sample Holding Pulse/2(HoldDataTicks_Value)

== system Navigation_KF_Lib/Navigation/CheckSum Pre-Processing/TempFilter/Process Raw Mag Data ==
  note: magnetometer[ 0 ] = - ( float ) navdata.mx ;
      | magnetometer[ 1 ] = ( float ) navdata.my ;
      | magnetometer[ 2 ] = - ( float ) navdata.mz ;
      | const float Sensitivity[ 3 ] = { 0.0071492608 , 0.0070882491 , 0.0074057781 } ;
      | const float Neutral[ 3 ] = { 118.0 , - 65.0 , 110.0 } ;
  Magnetometer : Inport
  Bias : Constant  Value=[ 118.0, -65.0, 110.0 ]
  Sum : Sum  Inputs=|+-
  postGain : Gain  Gain=[0.0071492608, 0.0070882491, 0.0074057781]
  preGain : Gain  Gain=[-1 1 -1]
  ProcessedData : Outport
  wires:
  postGain/1 -> ProcessedData/1
  Magnetometer/1 -> preGain/1
  Sum/1 -> postGain/1
  preGain/1 -> Sum/1
  Bias/1 -> Sum/2

== system Navigation_KF_Lib/Navigation/CheckSum Pre-Processing/Ultrasound Processing/CheckSum Correction ==
  CalculatedData : Inport
  CheckSumFlag : Inport  Port=2
  Holding Value : Inport  Port=3
  Compare To Zero : simulink/Logic and Bit Operations/Compare To Zero  relop=>  OutDataTypeStr=boolean
  Delay : Delay  DelayLength=3  InitialCondition=0
  Generate Sample Holding Pulse : Subsystem
  "If True, we have good data, If false, we have bad data, With bad data, use previous good data from N samples ago and hold it on that value for M samples" : Switch  Criteria=u2 > Threshold
  Invert Logic : Logic  Operator=NOT  AllPortsSameDT=off  OutDataTypeStr=boolean
  Logical Operator1 : Logic  Operator=NOT  AllPortsSameDT=off  OutDataTypeStr=boolean
  Pre-Processed Height : Outport
  wires:
  CheckSumFlag/1 -> Compare To Zero/1
  CalculatedData/1 -> "If True, we have good data, If false, we have bad data, With bad data, use previous good data from N samples ago and hold it on that value for M samples"/1
  "If True, we have good data, If false, we have bad data, With bad data, use previous good data from N samples ago and hold it on that value for M samples"/1 -> Pre-Processed Height/1, Delay/1
  Delay/1 -> "If True, we have good data, If false, we have bad data, With bad data, use previous good data from N samples ago and hold it on that value for M samples"/3
  Compare To Zero/1 -> Logical Operator1/1
  Generate Sample Holding Pulse/1(Hold_Data_Pulse) -> Invert Logic/1
  Logical Operator1/1 -> Generate Sample Holding Pulse/1(CheckSumFlag)
  Invert Logic/1 -> "If True, we have good data, If false, we have bad data, With bad data, use previous good data from N samples ago and hold it on that value for M samples"/2
  Holding Value/1 -> Generate Sample Holding Pulse/2(HoldDataTicks_Value)

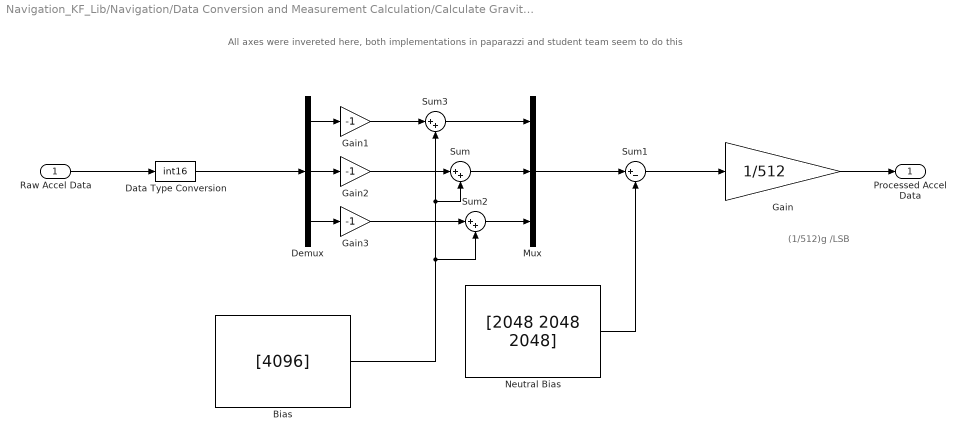
== system Navigation_KF_Lib/Navigation/Data Conversion and Measurement Calculation/Calculate Gravity Vector/Accelerometer Neutral Gain and Offset ==
  note: All axes were invereted here, both implementations in paparazzi and student team seem to do this
  note: (1/512)g /LSB
  Raw Accel Data : Inport
  Bias : Constant  Value=[4096]
  Data Type Conversion : DataTypeConversion  OutDataTypeStr=int16
  Demux : Demux  Outputs=3
  Gain : Gain  Gain=1/512
  Gain1 : Gain  Gain=-1  OutDataTypeStr=double
  Gain2 : Gain  Gain=-1  OutDataTypeStr=double
  Gain3 : Gain  Gain=-1  OutDataTypeStr=double
  Mux : Mux  Inputs=3
  Neutral Bias : Constant  Value=[2048 2048 2048]
  Sum : Sum  Inputs=|++
  Sum1 : Sum  Inputs=|+-
  Sum2 : Sum  Inputs=|++
  Sum3 : Sum  Inputs=|++
  Processed Accel Data : Outport
  wires:
  Sum1/1 -> Gain/1
  Gain/1 -> Processed Accel Data/1
  Mux/1 -> Sum1/1
  Neutral Bias/1 -> Sum1/2
  Raw Accel Data/1 -> Data Type Conversion/1
  Demux/1 -> Gain1/1
  Sum3/1 -> Mux/1
  Demux/2 -> Gain2/1
  Gain2/1 -> Sum/1
  Sum/1 -> Mux/2
  Demux/3 -> Gain3/1
  Gain3/1 -> Sum2/1
  Sum2/1 -> Mux/3
  Bias/1 -> Sum2/2, Sum/2, Sum3/2
  Data Type Conversion/1 -> Demux/1
  Gain1/1 -> Sum3/1

== system Navigation_KF_Lib/Navigation/Data Conversion and Measurement Calculation/Calculate Gravity Vector/Calibration_GainOffset ==
  Pre : Inport
  Accel_Calib_Gain : Constant  Value=[Accel_Calib_Gain.Gain_X Accel_Calib_Gain.Gain_Y Accel_Calib_Gain.Gain_Z]
      settings: AttributesFormatString=%<Value>
  Accel_Calib_Offset : Constant  Value="[Accel_Calib_Offset.Gain_X  Accel_Calib_Offset.Gain_Y  Accel_Calib_Offset.Gain_Z]"
      settings: AttributesFormatString=%<Value>
  Gain : Gain  Gain=-1  OutDataTypeStr=Inherit: Same as input
  Multiply : Product  Inputs=*/
  Sum : Sum  Inputs=|+-
  Post : Outport
  wires:
  Multiply/1 -> Post/1
  Accel_Calib_Offset/1 -> Sum/2
  Sum/1 -> Multiply/1
  Pre/1 -> Sum/1
  Accel_Calib_Gain/1 -> Gain/1
  Gain/1 -> Multiply/2

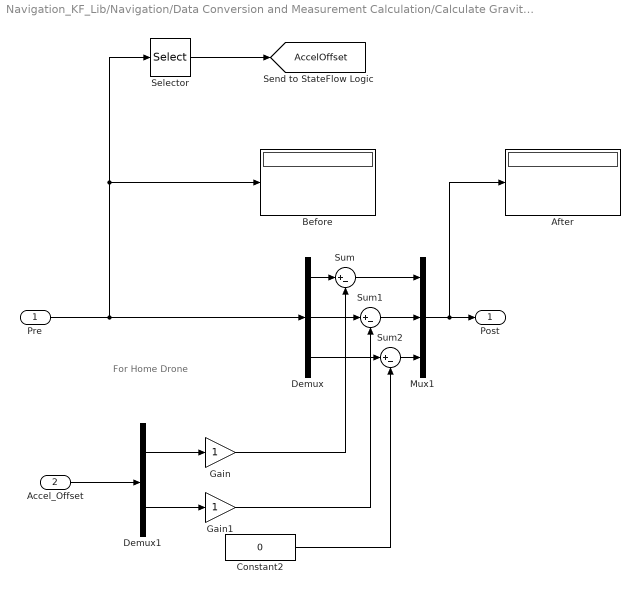
== system Navigation_KF_Lib/Navigation/Data Conversion and Measurement Calculation/Calculate Gravity Vector/InitialCondition_Offset ==
  note: For Home Drone
  Pre : Inport
  Accel_Offset : Inport  Port=2
  After : Display
  Before : Display
  Constant2 : Constant  Value=0
  Demux : Demux  Outputs=3
  Demux1 : Demux  Outputs=2
  Gain : Gain
  Gain1 : Gain
  Mux1 : Mux  Inputs=3
  Selector : Selector  InputPortWidth=3  IndexOptions=Index vector (dialog)  Indices=[1 2]  OutputSizes=1
  Sum : Sum  Inputs=|+-
  Sum1 : Sum  Inputs=|+-
  Sum2 : Sum  Inputs=|+-
  Post : Outport
  tag scope: AccelOffset=global
  wires:
  Sum/1 -> Mux1/1
  Sum2/1 -> Mux1/3
  Demux/3 -> Sum2/1
  Sum1/1 -> Mux1/2
  Demux/1 -> Sum/1
  Demux/2 -> Sum1/1
  Mux1/1 -> Post/1, After/1
  Accel_Offset/1 -> Demux1/1
  Demux1/1 -> Gain/1
  Demux1/2 -> Gain1/1
  Pre/1 -> Demux/1, Selector/1, Before/1
  Selector/1 -> [AccelOffset]
  Gain/1 -> Sum/2
  Gain1/1 -> Sum1/2
  Constant2/1 -> Sum2/2

== system Navigation_KF_Lib/Navigation/Data Conversion and Measurement Calculation/Calculate Gravity Vector/Low Pass Filter ==
  Offset Accel : Inport
  Add : Sum
  Gain : Gain  Gain=0.8
  Gain1 : Gain  Gain=0.2
  Unit Delay : UnitDelay  SampleTime=-1
  Filtered Accel : Outport
  wires:
  Unit Delay/1 -> Gain/1
  Gain1/1 -> Add/1
  Gain/1 -> Add/2
  Add/1 -> Unit Delay/1, Filtered Accel/1
  Offset Accel/1 -> Gain1/1

== system Navigation_KF_Lib/Navigation/Data Conversion and Measurement Calculation/Calibration_Scale_and_Offset/Process Raw Mag Data ==
  Magnetometer : Inport
  Process Raw Mag Data (Home_330453) : Subsystem  VariantControl=TempVariantA
  Process Raw Mag Data (Work_255725) : Subsystem  VariantControl=TempVariantB
  MagVector : Outport

== system Navigation_KF_Lib/Navigation/Data Conversion and Measurement Calculation/Remove Offset/Process Raw Rate Gyro Data ==
  note: const float Sensitivity[ 3 ] = { 0.0609 , 0.0609 , 0.0609 } ;
      | const float Neutral[ 3 ] = { 0.0 , 0.0 , 0.0 } ;
      | const int16_t Offset[ 3 ] = { - 73 , 14 , - 13 } ;
      | const int16_t Noises[ 3 ] = { 35 , 35 , 15 } ;
      |
      | int16_t vRaws[ 3 ] = {
      | Navdata :: IMU :: Gyroscope :: getRawX (),
      | Navdata :: IMU :: Gyroscope :: getRawY (),
      | Navdata :: IMU :: Gyroscope :: getRawZ ()
      | } ;
      |
      | gyroscope[i] = vRaws[i] * Gyroscope :: Sensitivity[i] * M_PI / 180.0 ;
  Raw Rate Gyro Data : Inport
  Gain : Gain  Gain=[0.0609, 0.0609, 0.0609]  ParamDataTypeStr=double
  Processed Data : Outport
  wires:
  Raw Rate Gyro Data/1 -> Gain/1
  Gain/1 -> Processed Data/1

== system Navigation_KF_Lib/Navigation/SL3D Visualization/Interchange Axes Mag for SL3D /Home Drone ==
  note: This comes close, however, it doesnt seem that the axis changes properly
      | ie: i rotate drone, the green dot follows it. This  tells me the Z-axis is not
      |  properly placed
  note: y
  note: x
  note: z
  In1 : Inport
  Demux1 : Demux  Outputs=3
  Gain : Gain  Gain=-1
  Gain1 : Gain
  Gain2 : Gain
  Mux2 : Mux  Inputs=3
  Out1 : Outport
  wires:
  Mux2/1 -> Out1/1
  In1/1 -> Demux1/1
  Demux1/3 -> Gain2/1
  Gain2/1 -> Mux2/2
  Demux1/1 -> Gain/1
  Gain/1 -> Mux2/3
  Demux1/2 -> Gain1/1
  Gain1/1 -> Mux2/1

== system Navigation_KF_Lib/Navigation/SL3D Visualization/Interchange Axes Mag for SL3D /Subsystem ==
  note: This comes close, however, it doesnt seem that the axis changes properly
      | ie: i rotate drone, the green dot follows it. This  tells me the Z-axis is not
      |  properly placed
  note: y
  note: x
  note: z
  In1 : Inport
  Demux1 : Demux  Outputs=3
  Gain : Gain
  Gain1 : Gain  Gain=-1
  Gain2 : Gain  Gain=-1
  Mux2 : Mux  Inputs=3
  Out1 : Outport
  wires:
  Demux1/1 -> Gain2/1
  Gain2/1 -> Mux2/2
  Gain/1 -> Mux2/3
  Gain1/1 -> Mux2/1
  Mux2/1 -> Out1/1
  Demux1/2 -> Gain1/1
  Demux1/3 -> Gain/1
  In1/1 -> Demux1/1

== system Navigation_KF_Lib/Navigation/SL3D Visualization/Interchange Axes Mag for SL3D /Work Drone ==
  note: This comes close, however, it doesnt seem that the axis changes properly
      | ie: i rotate drone, the green dot follows it. This  tells me the Z-axis is not
      |  properly placed
  note: y
  note: x
  note: z
  In1 : Inport
  Demux1 : Demux  Outputs=3
  Gain : Gain  Gain=-1
  Gain1 : Gain
  Gain2 : Gain
  Mux2 : Mux  Inputs=3
  Out1 : Outport
  wires:
  Mux2/1 -> Out1/1
  In1/1 -> Demux1/1
  Demux1/3 -> Gain2/1
  Gain2/1 -> Mux2/2
  Demux1/1 -> Gain/1
  Gain/1 -> Mux2/3
  Demux1/2 -> Gain1/1
  Gain1/1 -> Mux2/1

== system Navigation_KF_Lib/Navigation/SL3D Visualization/Interchange Axes Mag for SL3D /Work Drone - supposed work drone .. not really ==
  note: This comes close, however, it doesnt seem that the axis changes properly
      | ie: i rotate drone, the green dot follows it. This  tells me the Z-axis is not
      |  properly placed
  note: y
  note: x
  note: z
  In1 : Inport
  Demux1 : Demux  Outputs=3
  Gain : Gain  Gain=-1
  Gain1 : Gain
  Gain2 : Gain  Gain=-1
  Mux2 : Mux  Inputs=3
  Out1 : Outport
  wires:
  Mux2/1 -> Out1/1
  In1/1 -> Demux1/1
  Demux1/3 -> Gain2/1
  Gain2/1 -> Mux2/2
  Demux1/1 -> Gain/1
  Gain/1 -> Mux2/3
  Demux1/2 -> Gain1/1
  Gain1/1 -> Mux2/1

== system Navigation_KF_Lib/Navigation/CheckSum Pre-Processing/Accelerometer Processing/CheckSum Correction/Generate Sample Holding Pulse ==
  CheckSumFlag : Inport
  HoldDataTicks_Value : Inport  Port=2
  Chart : Stateflow chart  TreatAsAtomicUnit=on
  Constant2 : Constant
  Logical Operator1 : Logic  AllPortsSameDT=off  OutDataTypeStr=boolean
  Transition Logic Detection : Subsystem
  Hold_Data_Pulse : Outport
  wires:
  Constant2/1 -> Logical Operator1/1
  Logical Operator1/1 -> Hold_Data_Pulse/1
  Chart/1(output) -> Logical Operator1/2
  Transition Logic Detection/1(Transition Detect) -> Chart/1(if_transition)
  CheckSumFlag/1 -> Transition Logic Detection/1(Input)
  HoldDataTicks_Value/1 -> Chart/2(HoldDataTicks)

== system Navigation_KF_Lib/Navigation/CheckSum Pre-Processing/Magnetometer/CheckSum Correction/Generate Sample Holding Pulse ==
  CheckSumFlag : Inport
  HoldDataTicks_Value : Inport  Port=2
  Chart : Stateflow chart  TreatAsAtomicUnit=on
  Constant2 : Constant
  Logical Operator1 : Logic  AllPortsSameDT=off  OutDataTypeStr=boolean
  Transition Logic Detection : Subsystem
  Hold_Data_Pulse : Outport
  wires:
  Constant2/1 -> Logical Operator1/1
  Logical Operator1/1 -> Hold_Data_Pulse/1
  Chart/1(output) -> Logical Operator1/2
  Transition Logic Detection/1(Transition Detect) -> Chart/1(if_transition)
  CheckSumFlag/1 -> Transition Logic Detection/1(Input)
  HoldDataTicks_Value/1 -> Chart/2(HoldDataTicks)

== system Navigation_KF_Lib/Navigation/CheckSum Pre-Processing/RateGyro Processing/CheckSum Correction/Generate Sample Holding Pulse ==
  CheckSumFlag : Inport
  HoldDataTicks_Value : Inport  Port=2
  Chart : Stateflow chart  TreatAsAtomicUnit=on
  Constant2 : Constant
  Logical Operator1 : Logic  AllPortsSameDT=off  OutDataTypeStr=boolean
  Transition Logic Detection : Subsystem
  Hold_Data_Pulse : Outport
  wires:
  Constant2/1 -> Logical Operator1/1
  Logical Operator1/1 -> Hold_Data_Pulse/1
  Chart/1(output) -> Logical Operator1/2
  Transition Logic Detection/1(Transition Detect) -> Chart/1(if_transition)
  CheckSumFlag/1 -> Transition Logic Detection/1(Input)
  HoldDataTicks_Value/1 -> Chart/2(HoldDataTicks)

== system Navigation_KF_Lib/Navigation/CheckSum Pre-Processing/TempFilter/CheckSum Correction/Generate Sample Holding Pulse ==
  CheckSumFlag : Inport
  HoldDataTicks_Value : Inport  Port=2
  Chart : Stateflow chart  TreatAsAtomicUnit=on
  Constant2 : Constant
  Logical Operator1 : Logic  AllPortsSameDT=off  OutDataTypeStr=boolean
  Transition Logic Detection : Subsystem
  Hold_Data_Pulse : Outport
  wires:
  Constant2/1 -> Logical Operator1/1
  Logical Operator1/1 -> Hold_Data_Pulse/1
  Chart/1(output) -> Logical Operator1/2
  Transition Logic Detection/1(Transition Detect) -> Chart/1(if_transition)
  CheckSumFlag/1 -> Transition Logic Detection/1(Input)
  HoldDataTicks_Value/1 -> Chart/2(HoldDataTicks)

== system Navigation_KF_Lib/Navigation/CheckSum Pre-Processing/Ultrasound Processing/CheckSum Correction/Generate Sample Holding Pulse ==
  CheckSumFlag : Inport
  HoldDataTicks_Value : Inport  Port=2
  Chart : Stateflow chart  TreatAsAtomicUnit=on
  Constant2 : Constant
  Logical Operator1 : Logic  AllPortsSameDT=off  OutDataTypeStr=boolean
  Transition Logic Detection : Subsystem
  Hold_Data_Pulse : Outport
  wires:
  Constant2/1 -> Logical Operator1/1
  Logical Operator1/1 -> Hold_Data_Pulse/1
  Chart/1(output) -> Logical Operator1/2
  Transition Logic Detection/1(Transition Detect) -> Chart/1(if_transition)
  CheckSumFlag/1 -> Transition Logic Detection/1(Input)
  HoldDataTicks_Value/1 -> Chart/2(HoldDataTicks)

== system Navigation_KF_Lib/Navigation/Data Conversion and Measurement Calculation/Calibration_Scale_and_Offset/Process Raw Mag Data/Process Raw Mag Data (Home_330453) ==
  note: magnetometer[ 0 ] = - ( float ) navdata.mx ;
      | magnetometer[ 1 ] = ( float ) navdata.my ;
      | magnetometer[ 2 ] = - ( float ) navdata.mz ;
      | const float Sensitivity[ 3 ] = { 0.0071492608 , 0.0070882491 , 0.0074057781 } ;
      | const float Neutral[ 3 ] = { 118.0 , - 65.0 , 110.0 } ;
  Magnetometer : Inport
  Bias : Constant  Commented=on  Value=[-23 4.3 1.44]
  Constant : Constant  Value=[Mag_Calib_Offset_Vector.Gain_X Mag_Calib_Offset_Vector.Gain_Y Mag_Calib_Offset_Vector.Gain_Z]
      settings: AttributesFormatString=%<Value>
  Constant1 : Constant  Value=[Mag_Calib_Gain_Vector.Gain_X Mag_Calib_Gain_Vector.Gain_Y Mag_Calib_Gain_Vector.Gain_Z]
      settings: AttributesFormatString=%<Value>
  Divide : Product  Inputs=/*
  Sum : Sum  Inputs=|+-
  postGain : Gain  Commented=on  Gain=1./[187 163 139]
  MagVector : Outport
  wires:
  Divide/1 -> MagVector/1
  Constant/1 -> Sum/2
  Magnetometer/1 -> Sum/1
  Sum/1 -> Divide/2
  Constant1/1 -> Divide/1

== system Navigation_KF_Lib/Navigation/Data Conversion and Measurement Calculation/Calibration_Scale_and_Offset/Process Raw Mag Data/Process Raw Mag Data (Work_255725) ==
  note: magnetometer[ 0 ] = - ( float ) navdata.mx ;
      | magnetometer[ 1 ] = ( float ) navdata.my ;
      | magnetometer[ 2 ] = - ( float ) navdata.mz ;
      | const float Sensitivity[ 3 ] = { 0.0071492608 , 0.0070882491 , 0.0074057781 } ;
      | const float Neutral[ 3 ] = { 118.0 , - 65.0 , 110.0 } ;
  note: 158 145 136
  Magnetometer : Inport
  Bias : Constant  Value=[2.93 18.9 77.5]
  Low Pass Filter1 : Subsystem  Commented=through
      mask Display: disp(['Elliptic Filter with 20 Hz corner', '\n', '44 dB stopband.'])
  Sum : Sum  Inputs=|+-
  postGain : Gain  Gain=1./[167 135 132]
  preGain : Gain  Commented=through  Gain=[1 1 1]
  MagVector : Outport
  wires:
  Low Pass Filter1/1(Output) -> MagVector/1
  Bias/1 -> Sum/2
  preGain/1 -> Sum/1
  Sum/1 -> postGain/1
  Magnetometer/1 -> preGain/1
  postGain/1 -> Low Pass Filter1/1(Input)

== system Navigation_KF_Lib/Navigation/CheckSum Pre-Processing/Accelerometer Processing/CheckSum Correction/Generate Sample Holding Pulse/Transition Logic Detection ==
  Input : Inport
  Constant : Constant  Value=0
  Constant1 : Constant
  Logical Operator : Logic  AllPortsSameDT=off  OutDataTypeStr=boolean
  Relational Operator : RelationalOperator  Operator===  OutDataTypeStr=boolean
  Relational Operator1 : RelationalOperator  Operator===  OutDataTypeStr=boolean
  Unit Delay : UnitDelay  SampleTime=-1
  Transition Detect : Outport
  wires:
  Relational Operator1/1 -> Logical Operator/1
  Unit Delay/1 -> Relational Operator/1
  Input/1 -> Relational Operator1/2, Unit Delay/1
  Relational Operator/1 -> Logical Operator/2
  Constant/1 -> Relational Operator/2
  Constant1/1 -> Relational Operator1/1
  Logical Operator/1 -> Transition Detect/1  "Transition_Detect"

== system Navigation_KF_Lib/Navigation/CheckSum Pre-Processing/Magnetometer/CheckSum Correction/Generate Sample Holding Pulse/Transition Logic Detection ==
  Input : Inport
  Constant : Constant  Value=0
  Constant1 : Constant
  Logical Operator : Logic  AllPortsSameDT=off  OutDataTypeStr=boolean
  Relational Operator : RelationalOperator  Operator===  OutDataTypeStr=boolean
  Relational Operator1 : RelationalOperator  Operator===  OutDataTypeStr=boolean
  Unit Delay : UnitDelay  SampleTime=-1
  Transition Detect : Outport
  wires:
  Relational Operator1/1 -> Logical Operator/1
  Unit Delay/1 -> Relational Operator/1
  Input/1 -> Relational Operator1/2, Unit Delay/1
  Relational Operator/1 -> Logical Operator/2
  Constant/1 -> Relational Operator/2
  Constant1/1 -> Relational Operator1/1
  Logical Operator/1 -> Transition Detect/1  "Transition_Detect"

== system Navigation_KF_Lib/Navigation/CheckSum Pre-Processing/RateGyro Processing/CheckSum Correction/Generate Sample Holding Pulse/Transition Logic Detection ==
  Input : Inport
  Constant : Constant  Value=0
  Constant1 : Constant
  Logical Operator : Logic  AllPortsSameDT=off  OutDataTypeStr=boolean
  Relational Operator : RelationalOperator  Operator===  OutDataTypeStr=boolean
  Relational Operator1 : RelationalOperator  Operator===  OutDataTypeStr=boolean
  Unit Delay : UnitDelay  SampleTime=-1
  Transition Detect : Outport
  wires:
  Relational Operator1/1 -> Logical Operator/1
  Unit Delay/1 -> Relational Operator/1
  Input/1 -> Relational Operator1/2, Unit Delay/1
  Relational Operator/1 -> Logical Operator/2
  Constant/1 -> Relational Operator/2
  Constant1/1 -> Relational Operator1/1
  Logical Operator/1 -> Transition Detect/1  "Transition_Detect"

== system Navigation_KF_Lib/Navigation/CheckSum Pre-Processing/TempFilter/CheckSum Correction/Generate Sample Holding Pulse/Transition Logic Detection ==
  Input : Inport
  Constant : Constant  Value=0
  Constant1 : Constant
  Logical Operator : Logic  AllPortsSameDT=off  OutDataTypeStr=boolean
  Relational Operator : RelationalOperator  Operator===  OutDataTypeStr=boolean
  Relational Operator1 : RelationalOperator  Operator===  OutDataTypeStr=boolean
  Unit Delay : UnitDelay  SampleTime=-1
  Transition Detect : Outport
  wires:
  Relational Operator1/1 -> Logical Operator/1
  Unit Delay/1 -> Relational Operator/1
  Input/1 -> Relational Operator1/2, Unit Delay/1
  Relational Operator/1 -> Logical Operator/2
  Constant/1 -> Relational Operator/2
  Constant1/1 -> Relational Operator1/1
  Logical Operator/1 -> Transition Detect/1  "Transition_Detect"

== system Navigation_KF_Lib/Navigation/CheckSum Pre-Processing/Ultrasound Processing/CheckSum Correction/Generate Sample Holding Pulse/Transition Logic Detection ==
  Input : Inport
  Constant : Constant  Value=0
  Constant1 : Constant
  Logical Operator : Logic  AllPortsSameDT=off  OutDataTypeStr=boolean
  Relational Operator : RelationalOperator  Operator===  OutDataTypeStr=boolean
  Relational Operator1 : RelationalOperator  Operator===  OutDataTypeStr=boolean
  Unit Delay : UnitDelay  SampleTime=-1
  Transition Detect : Outport
  wires:
  Relational Operator1/1 -> Logical Operator/1
  Unit Delay/1 -> Relational Operator/1
  Input/1 -> Relational Operator1/2, Unit Delay/1
  Relational Operator/1 -> Logical Operator/2
  Constant/1 -> Relational Operator/2
  Constant1/1 -> Relational Operator1/1
  Logical Operator/1 -> Transition Detect/1  "Transition_Detect"
